simulink model "StopConditions_UnitTest"  (R2018b)
settings: Solver=FixedStepDiscrete  StartTime=0.0  StopTime=3000  FixedStep=1.0  RelTol=1e-3  EnableMultiTasking=on
libraries: simulink x1, StopConditionsBlock x1
settings Model: Creator=ri18384  LastModifiedBy=BI28030
settings DataIOCC: LimitDataPoints=on  SaveFormat=Array
settings OptimizationCC: ExpressionDepthLimit=2147483647  LifeSpan=inf
settings DebuggingCC: UnderspecifiedInitializationDetection=Classic  MergeDetectMultiDrivingBlocksExec=none  SolverPrmCheckMsg=warning  StateNameClashWarn=warning  SFUnexpectedBacktrackingDiag=warning  SFNoUnconditionalDefaultTransitionDiag=warning  SFExecutionAtInitializationDiag=none
settings HardwareCC: ProdBitPerPointer=32  ProdBitPerSizeT=32  ProdBitPerPtrDiffT=32  ProdLargestAtomicFloat=None  ProdIntDivRoundTo=Undefined  ProdEndianess=Unspecified  ProdWordSize=32  ProdHWDeviceType=32-bit Generic
settings ModelReferenceCC: PropagateSignalLabelsOutOfModel=off
settings SFSimCC: SimUseLocalCustomCode=off
settings RTWCC: RTWUseLocalCustomCode=off
settings CodeAppCC: StateflowObjectComments=on
settings GRTTargetCC: TargetLangStandard=C89/C90 (ANSI)  GeneratePreprocessorConditionals=Disable all
settings ConfigComp: CovMetricSettings=dw  CovHtmlReporting=on  CovSaveCumulativeToWorkspaceVar=on  CovSaveSingleToWorkspaceVar=on  CovExternalEMLEnable=off

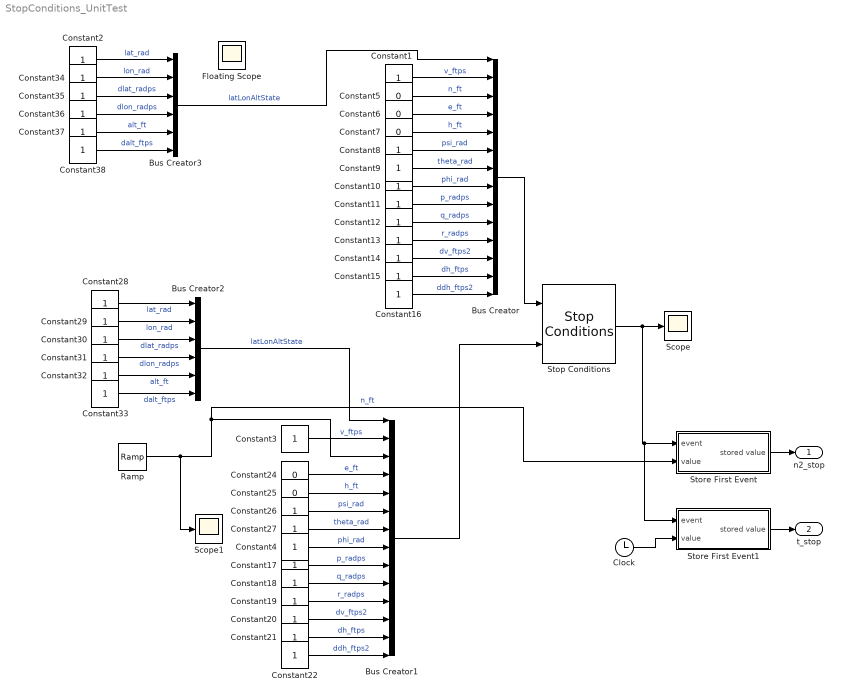
== system StopConditions_UnitTest ==
  Bus Creator : BusCreator  Inputs=14  OutDataTypeStr=Bus: AircraftState
  Bus Creator1 : BusCreator  Inputs=14  OutDataTypeStr=Bus: AircraftState
  Bus Creator2 : BusCreator  Inputs=6
  Bus Creator3 : BusCreator  Inputs=6
  Clock : Clock
  Constant{1..4,8..22,26..38} (32 alike) : Constant
  Constant{5..7,24..25} (5 alike) : Constant  Value=0
  Ramp : simulink/Sources/Ramp  slope=-1  start=0  InitialOutput=1100
  Scope : Scope
  Scope1 : Scope
  Stop Conditions : StopConditionsBlock/Stop Conditions  range_limit_ft=stop_range_ft  altitude_limit_ft=stop_altitude_ft
  Store First Event : Subsystem
  Store First Event1 : Subsystem
  n2_stop : Outport
  t_stop : Outport  Port=2
  Floating Scope : Scope
  wires:
  Bus Creator/1 -> Stop Conditions/1
  Bus Creator3/1 -> Bus Creator/1  "latLonAltState"
  Constant1/1 -> Bus Creator/2  "v_ftps"
  Stop Conditions/1 -> Store First Event1/1(event), Store First Event/1(event), Scope/1
  Constant5/1 -> Bus Creator/3  "n_ft"
  Constant6/1 -> Bus Creator/4  "e_ft"
  Constant7/1 -> Bus Creator/5  "h_ft"
  Constant8/1 -> Bus Creator/6  "psi_rad"
  Constant9/1 -> Bus Creator/7  "theta_rad"
  Constant10/1 -> Bus Creator/8  "phi_rad"
  Constant11/1 -> Bus Creator/9  "p_radps"
  Constant12/1 -> Bus Creator/10  "q_radps"
  Constant13/1 -> Bus Creator/11  "r_radps"
  Constant14/1 -> Bus Creator/12  "dv_ftps2"
  Constant15/1 -> Bus Creator/13  "dh_ftps"
  Constant16/1 -> Bus Creator/14  "ddh_ftps2"
  Bus Creator2/1 -> Bus Creator1/1  "latLonAltState"
  Constant3/1 -> Bus Creator1/2  "v_ftps"
  Ramp/1 -> Scope1/1, Store First Event/2(value), Bus Creator1/3  "n_ft"
  Constant24/1 -> Bus Creator1/4  "e_ft"
  Constant25/1 -> Bus Creator1/5  "h_ft"
  Constant26/1 -> Bus Creator1/6  "psi_rad"
  Constant27/1 -> Bus Creator1/7  "theta_rad"
  Constant4/1 -> Bus Creator1/8  "phi_rad"
  Constant17/1 -> Bus Creator1/9  "p_radps"
  Constant18/1 -> Bus Creator1/10  "q_radps"
  Constant19/1 -> Bus Creator1/11  "r_radps"
  Constant20/1 -> Bus Creator1/12  "dv_ftps2"
  Constant21/1 -> Bus Creator1/13  "dh_ftps"
  Constant22/1 -> Bus Creator1/14  "ddh_ftps2"
  Bus Creator1/1 -> Stop Conditions/2
  Constant28/1 -> Bus Creator2/1  "lat_rad"
  Constant29/1 -> Bus Creator2/2  "lon_rad"
  Constant30/1 -> Bus Creator2/3  "dlat_radps"
  Constant31/1 -> Bus Creator2/4  "dlon_radps"
  Constant32/1 -> Bus Creator2/5  "alt_ft"
  Constant33/1 -> Bus Creator2/6  "dalt_ftps"
  Constant2/1 -> Bus Creator3/1  "lat_rad"
  Constant34/1 -> Bus Creator3/2  "lon_rad"
  Constant35/1 -> Bus Creator3/3  "dlat_radps"
  Constant36/1 -> Bus Creator3/4  "dlon_radps"
  Constant37/1 -> Bus Creator3/5  "alt_ft"
  Constant38/1 -> Bus Creator3/6  "dalt_ftps"
  Store First Event/1(stored value) -> n2_stop/1
  Clock/1 -> Store First Event1/2(value)
  Store First Event1/1(stored value) -> t_stop/1

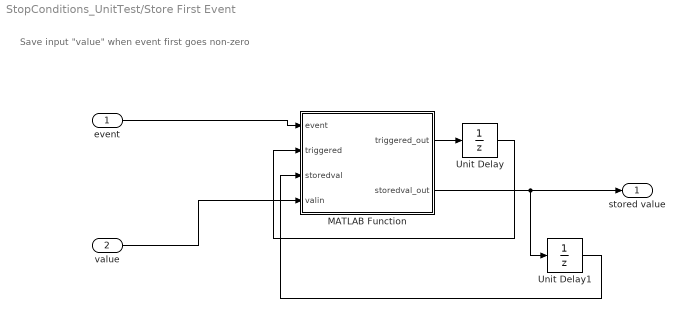
== system StopConditions_UnitTest/Store First Event ==
  note: Save input "value" when event first goes non-zero
  event : Inport
  value : Inport  Port=2
  MATLAB Function : MATLAB Function  TreatAsAtomicUnit=on
  Unit Delay : UnitDelay  SampleTime=-1
  Unit Delay1 : UnitDelay  SampleTime=-1
  stored value : Outport
  wires:
  event/1 -> MATLAB Function/1(event)
  MATLAB Function/1(triggered_out) -> Unit Delay/1
  Unit Delay/1 -> MATLAB Function/2(triggered)
  MATLAB Function/2(storedval_out) -> Unit Delay1/1, stored value/1
  Unit Delay1/1 -> MATLAB Function/3(storedval)
  value/1 -> MATLAB Function/4(valin)

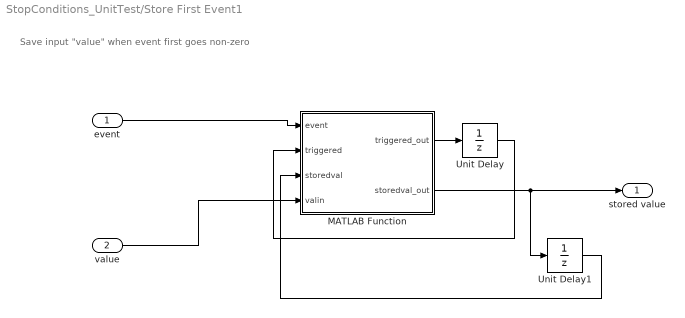
== system StopConditions_UnitTest/Store First Event1 ==
  note: Save input "value" when event first goes non-zero
  event : Inport
  value : Inport  Port=2
  MATLAB Function : MATLAB Function  TreatAsAtomicUnit=on
  Unit Delay : UnitDelay  SampleTime=-1
  Unit Delay1 : UnitDelay  SampleTime=-1
  stored value : Outport
  wires:
  event/1 -> MATLAB Function/1(event)
  MATLAB Function/1(triggered_out) -> Unit Delay/1
  Unit Delay/1 -> MATLAB Function/2(triggered)
  MATLAB Function/2(storedval_out) -> Unit Delay1/1, stored value/1
  Unit Delay1/1 -> MATLAB Function/3(storedval)
  value/1 -> MATLAB Function/4(valin)

== matlab function StopConditions_UnitTest/Store First Event1/MATLAB Function ==
  data: event input; triggered_out output; triggered input; storedval input; valin input; storedval_out output
function [triggered_out,storedval_out] = fcn(event,triggered,storedval,valin)

triggered_out = triggered;
storedval_out = storedval;

if( ~triggered )
    if( event~=0 )
        triggered_out=1;
        storedval_out=valin;
    end
end

== matlab function StopConditions_UnitTest/Store First Event/MATLAB Function ==
  data: event input; triggered_out output; triggered input; storedval input; valin input; storedval_out output
function [triggered_out,storedval_out] = fcn(event,triggered,storedval,valin)

triggered_out = triggered;
storedval_out = storedval;

if( ~triggered )
    if( event~=0 )
        triggered_out=1;
        storedval_out=valin;
    end
end
